simulink library "dragTurbineMantaNew_ul"  (R2020a)
settings: Solver=VariableStepAuto  StartTime=0.0  StopTime=10.0  RelTol=1e-3
undefined symbols (not defined in the file): rho, vcl
libraries: simulink x1, vrlib x1, vectorNormalizer_ul x1, localApparentWind_ul x1
settings Model: Creator=Ayaz  LastModifiedBy=JohnJr
settings DataIOCC: ReturnWorkspaceOutputs=off
settings DebuggingCC: ArithmeticOperatorsInVariantConditions=warning
settings SFSimCC: CustomCodeUndefinedFunction=UseInterfaceOnly

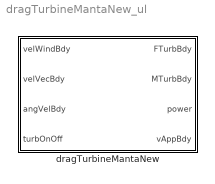
== system dragTurbineMantaNew_ul ==
  dragTurbineMantaNew : Subsystem  TreatAsAtomicUnit=on  mask{rho_fluid=rho, turb_struct=vcl.struct('OCT.turb')}
      mask prompts: rho_fluid "Fluid density"; turb_struct "Turbines structure"

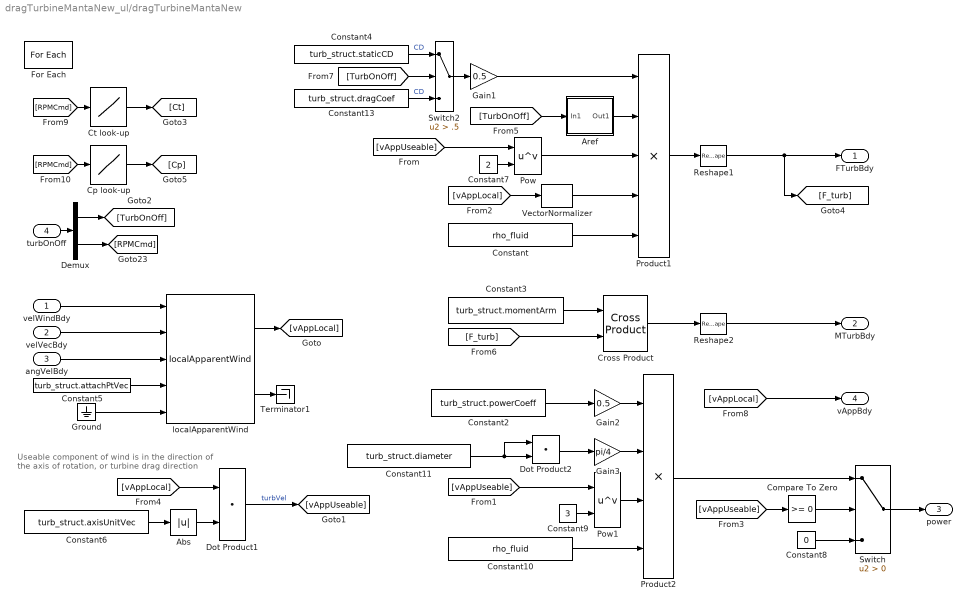
== system dragTurbineMantaNew_ul/dragTurbineMantaNew ==
  note: Useable component of wind is in the direction of
      | the axis of rotation, or turbine drag direction
  velWindBdy : Inport  Partition=on  PartitionDimension=2  PartitionWidth=1  PartitionOffset=0
  velVecBdy : Inport  Port=2
  angVelBdy : Inport  Port=3
  turbOnOff : Inport  Port=4
  Abs : Abs
  Aref : Subsystem
  Compare To Zero : simulink/Logic and Bit Operations/Compare To Zero  relop=>=  OutDataTypeStr=boolean
  Constant : Constant  Value=rho_fluid
  Constant10 : Constant  Value=rho_fluid
  Constant11 : Constant  Value=turb_struct.diameter  VectorParams1D=off
  Constant13 : Constant  Value=turb_struct.dragCoef
  Constant2 : Constant  Value=turb_struct.powerCoeff
  Constant3 : Constant  Value=turb_struct.momentArm
  Constant4 : Constant  Value=turb_struct.staticCD
  Constant5 : Constant  Value=turb_struct.attachPtVec
  Constant6 : Constant  Value=turb_struct.axisUnitVec
  Constant7 : Constant  Value=2
  Constant8 : Constant  Value=0
  Constant9 : Constant  Value=3
  Cp look-up : Lookup_n-D  NumberOfTableDimensions=1  BreakpointsForDimension1=[-5:5]  Table=tanh([-5:5])  InternalRulePriority=Speed  RndMeth=Simplest  InputSameDT=on
  Cross Product : vrlib/Utilities/Cross Product
  Ct look-up : Lookup_n-D  NumberOfTableDimensions=1  BreakpointsForDimension1=[-5:5]  Table=tanh([-5:5])  InternalRulePriority=Speed  RndMeth=Simplest  InputSameDT=on
  Demux : Demux  Outputs=2
  Dot Product1 : DotProduct  InputSameDT=on  OutDataTypeStr=Inherit: Inherit via internal rule
  Dot Product2 : DotProduct  InputSameDT=on  OutDataTypeStr=Inherit: Inherit via internal rule
  For Each : ForEach  DisableCoverage=on  IterateSubsysMaskParameter=off,on  SubsysMaskParameterIterationDimension=1,2
  Gain1 : Gain  Gain=0.5
  Gain2 : Gain  Gain=0.5
  Gain3 : Gain  Gain=pi/4
  Ground : Ground
  Pow : Math  Operator=pow  SignedPower=on  RndMeth=Zero  SaturateOnIntegerOverflow=on
  Pow1 : Math  Operator=pow  SignedPower=on  RndMeth=Zero  SaturateOnIntegerOverflow=on
  Product1 : Product  Inputs=5
  Product2 : Product  Inputs=4
  Reshape1 : Reshape  OutputDimensionality=Column vector (2-D)
  Reshape2 : Reshape  OutputDimensionality=Column vector (2-D)
  Switch : Switch  Criteria=u2 > Threshold
  Switch2 : Switch  Criteria=u2 > Threshold  Threshold=.5
  Terminator1 : Terminator
  "VectorNormalizer " : vectorNormalizer_ul/VectorNormalizer   SystemSampleTime=-1  Latency=0  AutoFrameSizeCalculation=off
  localApparentWind : localApparentWind_ul/localApparentWind  SystemSampleTime=-1  Latency=0  AutoFrameSizeCalculation=off
  FTurbBdy : Outport  PortDimensions=[3,1]  ConcatenationDimension=2  VectorParamsAs1DForOutWhenUnconnected=off
  MTurbBdy : Outport  Port=2  PortDimensions=[3,1]  ConcatenationDimension=2  VectorParamsAs1DForOutWhenUnconnected=off
  power : Outport  Port=3  PortDimensions=[1,1]  ConcatenationDimension=2  VectorParamsAs1DForOutWhenUnconnected=off
  vAppBdy : Outport  Port=4  PortDimensions=[3,1]  ConcatenationDimension=2  VectorParamsAs1DForOutWhenUnconnected=off
  wires:
  Gain3/1 -> Product2/2
  Constant11/1 -> Dot Product2/1, Dot Product2/2
  Dot Product2/1 -> Gain3/1
  [vAppUseable] -> Pow1/1
  [vAppLocal] -> Dot Product1/1
  Constant8/1 -> Switch/3
  [vAppUseable] -> Compare To Zero/1
  Compare To Zero/1 -> Switch/2
  Switch/1 -> power/1
  Constant7/1 -> Pow/2
  Pow/1 -> Product1/3
  Pow1/1 -> Product2/3
  Gain2/1 -> Product2/1
  Constant10/1 -> Product2/4
  Constant/1 -> Product1/5
  Gain1/1 -> Product1/1
  Dot Product1/1 -> [vAppUseable]  "turbVel"
  Constant9/1 -> Pow1/2
  "VectorNormalizer "/1 -> Product1/4
  [vAppUseable] -> Pow/1
  Constant6/1 -> Abs/1
  Constant5/1 -> localApparentWind/4
  localApparentWind/1 -> [vAppLocal]
  velWindBdy/1 -> localApparentWind/1
  angVelBdy/1 -> localApparentWind/3
  velVecBdy/1 -> localApparentWind/2
  Reshape2/1 -> MTurbBdy/1
  Reshape1/1 -> [F_turb], FTurbBdy/1
  [F_turb] -> Cross Product/2
  Constant3/1 -> Cross Product/1
  Product2/1 -> Switch/1
  Product1/1 -> Reshape1/1
  Cross Product/1 -> Reshape2/1
  Ground/1 -> localApparentWind/5
  localApparentWind/2 -> Terminator1/1
  Abs/1 -> Dot Product1/2
  [vAppLocal] -> "VectorNormalizer "/1
  Constant2/1 -> Gain2/1
  [vAppLocal] -> vAppBdy/1
  [TurbOnOff] -> Switch2/2
  Switch2/1 -> Gain1/1
  Constant4/1 -> Switch2/1  "CD"
  Constant13/1 -> Switch2/3  "CD"
  turbOnOff/1 -> Demux/1
  Demux/1 -> [TurbOnOff]
  Demux/2 -> [RPMCmd]
  [TurbOnOff] -> Aref/1(In1)
  Aref/1(Out1) -> Product1/2
  [RPMCmd] -> Ct look-up/1
  [RPMCmd] -> Cp look-up/1
  Ct look-up/1 -> [Ct]
  Cp look-up/1 -> [Cp]

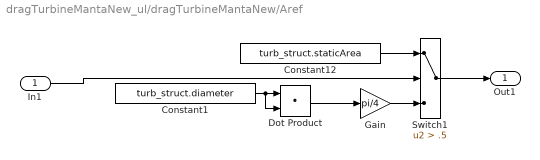
== system dragTurbineMantaNew_ul/dragTurbineMantaNew/Aref ==
  In1 : Inport
  Constant1 : Constant  Value=turb_struct.diameter  VectorParams1D=off
  Constant12 : Constant  Value=turb_struct.staticArea  VectorParams1D=off
  Dot Product : DotProduct  InputSameDT=on  OutDataTypeStr=Inherit: Inherit via internal rule
  Gain : Gain  Gain=pi/4
  Switch1 : Switch  Criteria=u2 > Threshold  Threshold=.5
  Out1 : Outport
  wires:
  Dot Product/1 -> Gain/1
  Constant1/1 -> Dot Product/2, Dot Product/1
  Switch1/1 -> Out1/1
  Gain/1 -> Switch1/3
  Constant12/1 -> Switch1/1
  In1/1 -> Switch1/2
